simulink model "B20_MR_DoS"  (R2020b)
settings: Solver=VariableStepAuto  StartTime=0.0  StopTime=tend  MaxStep=Ts  MinStep=0.001  RelTol=1.3e-2  EnableMultiTasking=on
values from neighbouring files (symbols this model uses):
  A1 = [-eta*eye(nloc)]    [B20_MR.m]    (also in B20_MR_DoS_design.m; B20_MR_Sin_Modificar.m; main.m)
  AA = 1.2    [B20_MR.m]    (also in B20_MR_DoS_design.m; B20_MR_Sin_Modificar.m; main.m)
  alph_a = 1.0872e07    (= 10872000)    [B20_MR.m]    (also in B20_MR_DoS_design.m; B20_MR_Sin_Modificar.m; main.m)
  alph_b = 4.9616e07    (= 49616000)    [B20_MR.m]    (also in B20_MR_DoS_design.m; B20_MR_Sin_Modificar.m; main.m)
  B1 = [eta*eye(nloc)]    [B20_MR.m]    (also in B20_MR_DoS_design.m; B20_MR_Sin_Modificar.m; main.m)
  BB = 300    [B20_MR.m]    (also in B20_MR_DoS_design.m; B20_MR_Sin_Modificar.m; main.m)
  c0_a = 4.40e2    (= 440)    [B20_MR.m]    (also in B20_MR_DoS_design.m; B20_MR_Sin_Modificar.m; main.m)
  c0_b = 44.0e2    (= 4400)    [B20_MR.m]    (also in B20_MR_DoS_design.m; B20_MR_Sin_Modificar.m; main.m)
  C1 = eye(nloc)    [B20_MR.m]    (also in B20_MR_DoS_design.m; B20_MR_Sin_Modificar.m; main.m)
  D1 = zeros(nloc,nloc)    [B20_MR.m]    (also in B20_MR_DoS_design.m; B20_MR_Sin_Modificar.m; main.m)
  DoS_p = ones(20,1)    [B20_MR.m]    (also in B20_MR_DoS_design.m; B20_MR_Sin_Modificar.m; main.m)
  DoS_s = ones(20,1)    [B20_MR.m]    (also in B20_MR_DoS_design.m; B20_MR_Sin_Modificar.m; main.m)
  EI = 1    [B20_MR.m]    (also in B20_MR_DoS_design.m = 0.7; B20_MR_Sin_Modificar.m; main.m = 0.4)
  GG = 300    [B20_MR.m]    (also in B20_MR_DoS_design.m; B20_MR_Sin_Modificar.m; main.m)
  K_lqr = lqr(A,B,Q,R)    [B20_MR.m]    (also in B20_MR_DoS_design.m = aux*K_lqr_un; B20_MR_Sin_Modificar.m; main.m = aux*K_lqr_un)
  Kdev = eye(20)    [B20_MR.m]    (also in B20_MR_DoS_design.m; B20_MR_Sin_Modificar.m; main.m)
  nloc = 20    [B20_MR.m]    (also in B20_MR_DoS_design.m; B20_MR_Sin_Modificar.m; main.m)
  Sys_con = ss(Ac,E,Cz,Dz)    [B20_MR.m]    (also in B20_MR_DoS_design.m = ss(A,[E B],C,D); B20_MR_Sin_Modificar.m = ss(A,[E B],C,D); main.m = ss(A,[E B],C,D))
  Sys_unc = ss(A_ref,E_ref,C_ref,DD_ref)    [B20_MR.m]    (also in B20_MR_DoS_design.m; B20_MR_Sin_Modificar.m; main.m)
  Ts = EQ.time(2)    [B20_MR.m]    (also in B20_MR_DoS_design.m; B20_MR_Sin_Modificar.m; main.m)
  Umax = 10    [B20_MR.m]    (also in B20_MR_DoS_design.m; B20_MR_Sin_Modificar.m; main.m)
libraries: dspindex x2
settings Model: Creator=drsoto  LastModifiedBy=ferch
settings SolverCC: ZeroCrossAlgorithm=Adaptive  AlgebraicLoopSolver=LineSearch
settings DataIOCC: ReturnWorkspaceOutputs=off
settings DebuggingCC: AlgebraicLoopMsg=none  IgnoredZcDiagnostic=none  ArithmeticOperatorsInVariantConditions=warning
settings ModelReferenceCC: PropagateSignalLabelsOutOfModel=off
settings SFSimCC: SimUseLocalCustomCode=off  CustomCodeUndefinedFunction=UseInterfaceOnly
settings RTWCC: RTWUseLocalCustomCode=off
settings CodeAppCC: StateflowObjectComments=on

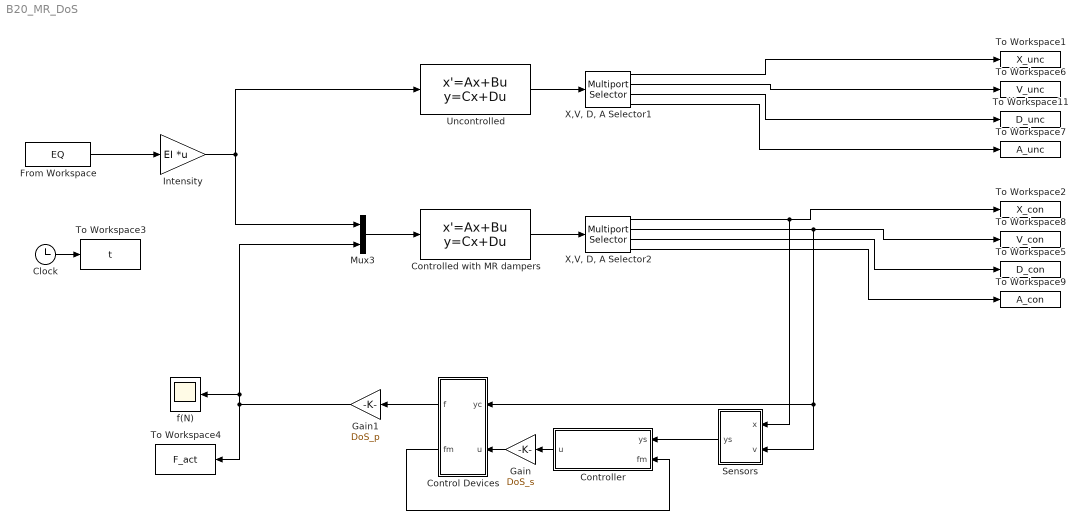
== system B20_MR_DoS ==
  Clock : Clock
  Control Devices : Subsystem
  Controlled with MR dampers : StateSpace  A=Sys_con.A  B=Sys_con.B  C=Sys_con.C  D=Sys_con.D  InitialCondition=0
  Controller : Subsystem
  From Workspace : FromWorkspace  VariableName=EQ  SampleTime=Ts
  Gain : Gain  Gain=DoS_s
  Gain1 : Gain  Gain=DoS_p
  Intensity : Gain  Gain=EI  Multiplication=Matrix(K*u)
  Mux3 : Mux  Inputs=2
  Sensors : Subsystem
  To Workspace1 : ToWorkspace  VariableName=X_unc  SampleTime=-1
  To Workspace11 : ToWorkspace  VariableName=D_unc  SampleTime=-1
  To Workspace2 : ToWorkspace  VariableName=X_con  SampleTime=-1
  To Workspace3 : ToWorkspace  VariableName=t  SampleTime=-1
      settings: Save2DSignal=2-D array (concatenate along first dimension)
  To Workspace4 : ToWorkspace  VariableName=F_act  SampleTime=-1
  To Workspace5 : ToWorkspace  VariableName=D_con  SampleTime=-1
  To Workspace6 : ToWorkspace  VariableName=V_unc  SampleTime=-1
  To Workspace7 : ToWorkspace  VariableName=A_unc  SampleTime=-1
  To Workspace8 : ToWorkspace  VariableName=V_con  SampleTime=-1
  To Workspace9 : ToWorkspace  VariableName=A_con  SampleTime=-1
  Uncontrolled : StateSpace  A=Sys_unc.A  B=Sys_unc.B  C=Sys_unc.C  D=Sys_unc.D  InitialCondition=0
  "X,V, D, A Selector1" : dspindex/Multiport Selector  rowsOrCols=Rows  idxCellArray={ 1:n,n+1:2*n,2*n+1:3*n,3*n+1:4*n}  idxErrMode=Clip Index
  "X,V, D, A Selector2" : dspindex/Multiport Selector  rowsOrCols=Rows  idxCellArray={ 1:n,n+1:2*n,2*n+1:3*n,3*n+1:4*n}  idxErrMode=Clip Index
  f(N) : Scope
  wires:
  Intensity/1 -> Uncontrolled/1, Mux3/1
  Uncontrolled/1 -> "X,V, D, A Selector1"/1
  From Workspace/1 -> Intensity/1
  Controlled with MR dampers/1 -> "X,V, D, A Selector2"/1
  Clock/1 -> To Workspace3/1
  "X,V, D, A Selector1"/2 -> To Workspace6/1
  Mux3/1 -> Controlled with MR dampers/1
  "X,V, D, A Selector1"/4 -> To Workspace7/1
  "X,V, D, A Selector1"/3 -> To Workspace11/1
  "X,V, D, A Selector2"/3 -> To Workspace5/1
  "X,V, D, A Selector2"/4 -> To Workspace9/1
  "X,V, D, A Selector1"/1 -> To Workspace1/1
  Control Devices/1(f) -> Gain1/1
  "X,V, D, A Selector2"/2 -> Control Devices/1(yc), Sensors/2(v), To Workspace8/1
  "X,V, D, A Selector2"/1 -> Sensors/1(x), To Workspace2/1
  Controller/1(u) -> Gain/1
  Sensors/1(ys) -> Controller/1(ys)
  Control Devices/2(fm) -> Controller/2(fm)
  Gain/1 -> Control Devices/2(u)
  Gain1/1 -> Mux3/2, f(N)/1, To Workspace4/1

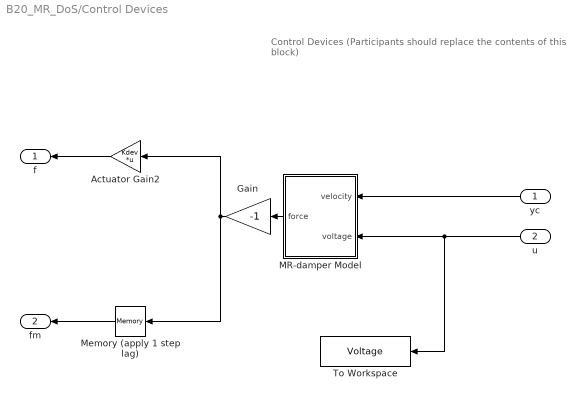
== system B20_MR_DoS/Control Devices ==
  note: Control Devices
      | (Participants should replace the contents of this block)
  yc : Inport
  u : Inport  Port=2
  Actuator Gain2 : Gain  Gain=Kdev  Multiplication=Matrix(K*u)  SaturateOnIntegerOverflow=on  OutDataTypeStr=Inherit: Same as input  ParamDataTypeStr=Inherit: Same as input
  Gain : Gain  Gain=-1  SaturateOnIntegerOverflow=on  OutDataTypeStr=Inherit: Same as input  ParamDataTypeStr=Inherit: Same as input
  MR-damper Model : Subsystem
  Memory (apply 1 step lag) : Memory  InheritSampleTime=on
  To Workspace : ToWorkspace  VariableName=Voltage  SampleTime=-1
  f : Outport  InitialOutput=0
  fm : Outport  Port=2  InitialOutput=0
  wires:
  u/1 -> To Workspace/1, MR-damper Model/2(voltage)
  yc/1 -> MR-damper Model/1(velocity)
  Gain/1 -> Actuator Gain2/1, Memory (apply 1 step lag)/1
  Actuator Gain2/1 -> f/1
  MR-damper Model/1(force) -> Gain/1
  Memory (apply 1 step lag)/1 -> fm/1

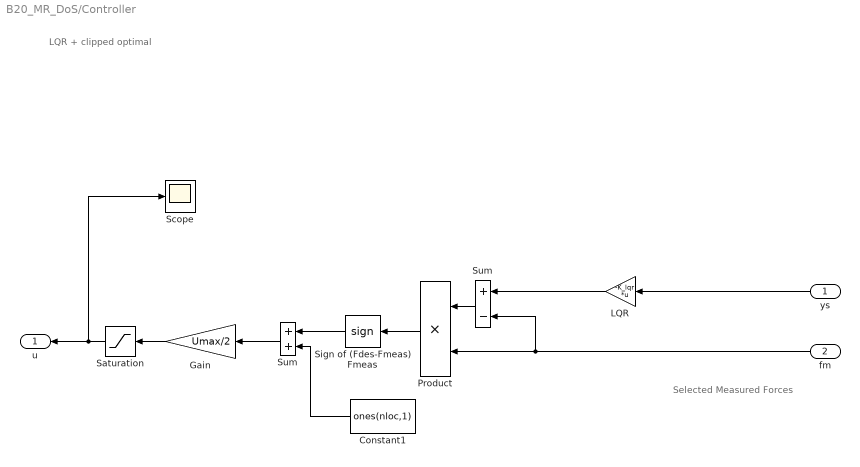
== system B20_MR_DoS/Controller ==
  note: LQR + clipped optimal
  note: Selected Measured Forces
  ys : Inport
  fm : Inport  Port=2
  Constant1 : Constant  Value=ones(nloc,1)
  Gain : Gain  Gain=Umax/2  SaturateOnIntegerOverflow=on  OutDataTypeStr=Inherit: Same as input  ParamDataTypeStr=Inherit: Same as input
  LQR : Gain  Gain=-K_lqr  Multiplication=Matrix(K*u)
  Product : Product  InputSameDT=on  SaturateOnIntegerOverflow=on  OutDataTypeStr=Inherit: Same as first input
  Saturation : Saturate  UpperLimit=Umax  LowerLimit=-Umax
  Scope : Scope
  Sign of (Fdes-Fmeas)Fmeas : Signum
  Sum : Sum  Inputs=+-  InputSameDT=on  SaturateOnIntegerOverflow=on  OutDataTypeStr=Inherit: Same as first input
  "Sum " : Sum  InputSameDT=on  SaturateOnIntegerOverflow=on  OutDataTypeStr=Inherit: Same as first input
  u : Outport
  wires:
  Saturation/1 -> Scope/1, u/1
  ys/1 -> LQR/1
  LQR/1 -> Sum/1
  Sign of (Fdes-Fmeas)Fmeas/1 -> "Sum "/1
  Product/1 -> Sign of (Fdes-Fmeas)Fmeas/1
  Sum/1 -> Product/1
  Constant1/1 -> "Sum "/2
  Gain/1 -> Saturation/1
  fm/1 -> Sum/2, Product/2
  "Sum "/1 -> Gain/1

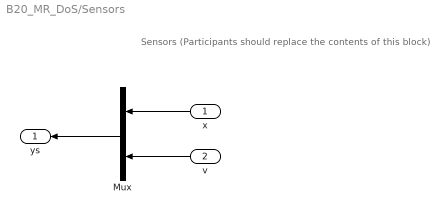
== system B20_MR_DoS/Sensors ==
  note: Sensors
      | (Participants should replace the contents of this block)
  x : Inport
  v : Inport  Port=2
  Mux : Mux  Inputs=2
  ys : Outport
  wires:
  Mux/1 -> ys/1
  x/1 -> Mux/1
  v/1 -> Mux/2

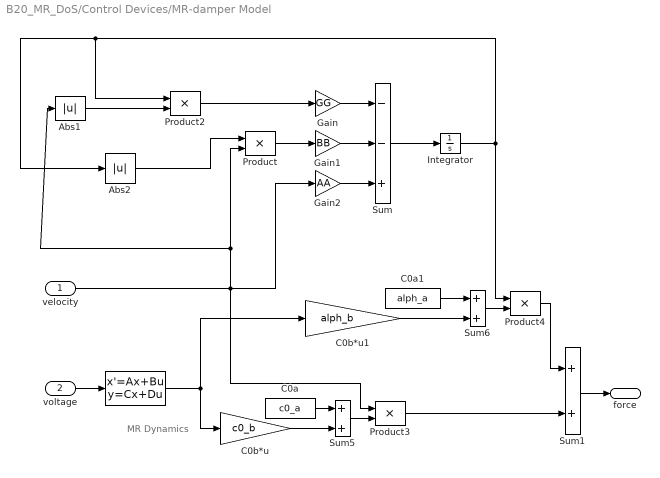
== system B20_MR_DoS/Control Devices/MR-damper Model ==
  note: MR Dynamics
  velocity : Inport
  voltage : Inport  Port=2
  " " : StateSpace  A=A1  B=B1  C=C1  D=D1  InitialCondition=0
  Abs1 : Abs  SaturateOnIntegerOverflow=on
  Abs2 : Abs  SaturateOnIntegerOverflow=on
  C0a : Constant  Value=c0_a
  C0a1 : Constant  Value=alph_a
  C0b*u : Gain  Gain=c0_b  SaturateOnIntegerOverflow=on  OutDataTypeStr=Inherit: Same as input  ParamDataTypeStr=Inherit: Same as input
  C0b*u1 : Gain  Gain=alph_b  SaturateOnIntegerOverflow=on  OutDataTypeStr=Inherit: Same as input  ParamDataTypeStr=Inherit: Same as input
  Gain : Gain  Gain=GG  SaturateOnIntegerOverflow=on  OutDataTypeStr=Inherit: Same as input  ParamDataTypeStr=Inherit: Same as input
  Gain1 : Gain  Gain=BB  SaturateOnIntegerOverflow=on  OutDataTypeStr=Inherit: Same as input  ParamDataTypeStr=Inherit: Same as input
  Gain2 : Gain  Gain=AA  SaturateOnIntegerOverflow=on  OutDataTypeStr=Inherit: Same as input  ParamDataTypeStr=Inherit: Same as input
  Integrator : Integrator
  Product{,2..4} (4 alike) : Product  InputSameDT=on  SaturateOnIntegerOverflow=on  OutDataTypeStr=Inherit: Same as first input
  Sum : Sum  Inputs=--+  InputSameDT=on  SaturateOnIntegerOverflow=on  OutDataTypeStr=Inherit: Same as first input
  Sum1 : Sum  InputSameDT=on  SaturateOnIntegerOverflow=on  OutDataTypeStr=Inherit: Same as first input
  Sum5 : Sum  InputSameDT=on  SaturateOnIntegerOverflow=on  OutDataTypeStr=Inherit: Same as first input
  Sum6 : Sum  InputSameDT=on  SaturateOnIntegerOverflow=on  OutDataTypeStr=Inherit: Same as first input
  force : Outport  InitialOutput=0
  wires:
  voltage/1 -> " "/1
  " "/1 -> C0b*u1/1, C0b*u/1
  Sum1/1 -> force/1
  Abs2/1 -> Product/1
  Product2/1 -> Gain/1
  Sum/1 -> Integrator/1
  Gain/1 -> Sum/1
  Gain1/1 -> Sum/2
  Gain2/1 -> Sum/3
  Product/1 -> Gain1/1
  Abs1/1 -> Product2/2
  velocity/1 -> Product/2, Abs1/1, Gain2/1, Product3/1
  Sum5/1 -> Product3/2
  C0a/1 -> Sum5/1
  C0b*u/1 -> Sum5/2
  Sum6/1 -> Product4/2
  C0a1/1 -> Sum6/1
  C0b*u1/1 -> Sum6/2
  Product3/1 -> Sum1/2
  Product4/1 -> Sum1/1
  Integrator/1 -> Abs2/1, Product2/1, Product4/1
